simulink model "Stability_model_VISUAL"  (R2023a)
settings: Solver=VariableStepAuto  StartTime=0.0  StopTime=1000  RelTol=1e-3
undefined symbols (not defined in the file): A, K, tau
settings Model: Creator=levir  LastModifiedBy=levir

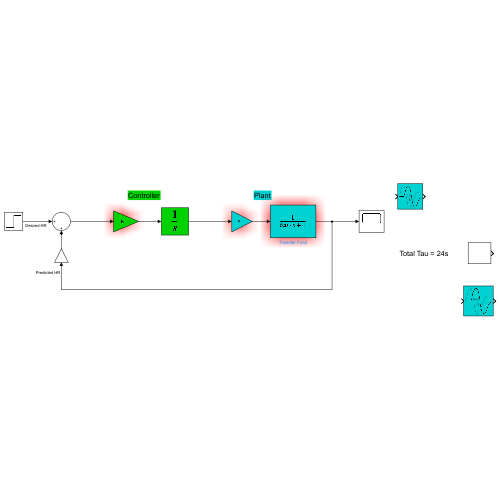
[thumbnail: Simulink's stored preview of the top-level diagram]
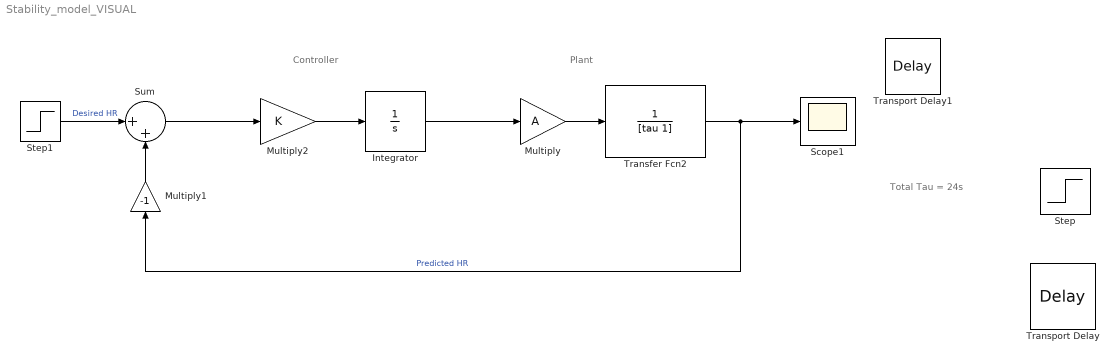
== system Stability_model_VISUAL ==
  note: Total Tau = 24s
  note: Controller
  note: Plant
  Integrator : Integrator
  Multiply : Gain  Gain=A
  Multiply1 : Gain  Gain=-1
  Multiply2 : Gain  Gain=K
  Scope1 : Scope
  Step : Step  Time=30  Before=100  After=170  SampleTime=0
  Step1 : Step  SampleTime=0
  Sum : Sum  Inputs=|++
  Transfer Fcn2 : TransferFcn  Denominator=[tau 1]
  Transport Delay : TransportDelay  DelayTime=24
  Transport Delay1 : TransportDelay  DelayTime=24
  wires:
  Step1/1 -> Sum/1  "Desired HR"
  Multiply/1 -> Transfer Fcn2/1
  Integrator/1 -> Multiply/1
  Sum/1 -> Multiply2/1
  Multiply2/1 -> Integrator/1
  Multiply1/1 -> Sum/2
  Transfer Fcn2/1 -> Multiply1/1, Scope1/1  "Predicted HR"
